simulink model "RateGyroUsingQuaternions"  (R2020b)
settings: Solver=VariableStepAuto  StartTime=0.0  StopTime=50  RelTol=1e-3
libraries: simulink_extras x1
settings Model: Creator=dariusmensah  LastModifiedBy=dariusmensah

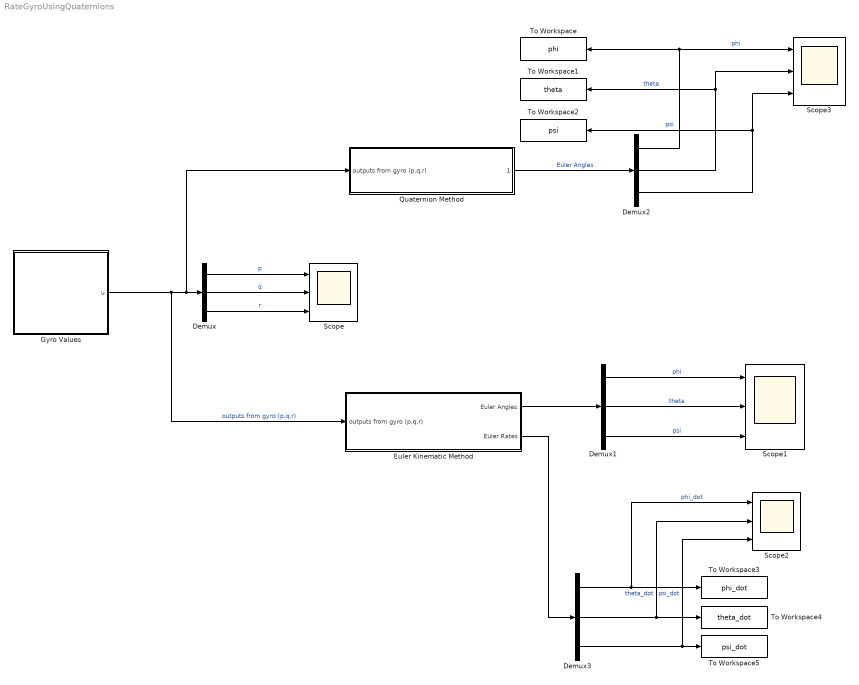
== system RateGyroUsingQuaternions ==
  Demux{,1..3} (4 alike) : Demux  Outputs=3
  Euler Kinematic Method : Subsystem
  Gyro Values : Subsystem
  Quaternion Method : Subsystem
  Scope{,1..3} (4 alike) : Scope  NumInputPorts=3
  To Workspace : ToWorkspace  VariableName=phi  SaveFormat=Structure With Time  SampleTime=-1
  To Workspace1 : ToWorkspace  VariableName=theta  SaveFormat=Structure With Time  SampleTime=-1
  To Workspace2 : ToWorkspace  VariableName=psi  SaveFormat=Structure With Time  SampleTime=-1
  To Workspace3 : ToWorkspace  VariableName=phi_dot  SaveFormat=Structure With Time  SampleTime=-1
  To Workspace4 : ToWorkspace  VariableName=theta_dot  SaveFormat=Structure With Time  SampleTime=-1
  To Workspace5 : ToWorkspace  VariableName=psi_dot  SaveFormat=Structure With Time  SampleTime=-1
  wires:
  Demux1/3 -> Scope1/3  "psi"
  Demux3/3 -> Scope2/3, To Workspace5/1  "psi_dot"
  Demux/3 -> Scope/3  "r"
  Gyro Values/1(u) -> Euler Kinematic Method/1(outputs from gyro (p,q,r)), Quaternion Method/1(outputs from gyro (p,q,r)), Demux/1  "outputs from gyro (p,q,r)"
  Demux/2 -> Scope/2  "q"
  Demux3/1 -> To Workspace3/1, Scope2/1  "phi_dot"
  Demux3/2 -> To Workspace4/1, Scope2/2  "theta_dot"
  Demux/1 -> Scope/1  "p"
  Demux1/1 -> Scope1/1  "phi"
  Demux1/2 -> Scope1/2  "theta"
  Quaternion Method/1(" ") -> Demux2/1  "Euler Angles"
  Demux2/1 -> To Workspace/1, Scope3/1  "phi"
  Demux2/2 -> Scope3/2, To Workspace1/1  "theta"
  Demux2/3 -> Scope3/3, To Workspace2/1  "psi"
  Euler Kinematic Method/1(Euler Angles) -> Demux1/1
  Euler Kinematic Method/2(Euler Rates) -> Demux3/1

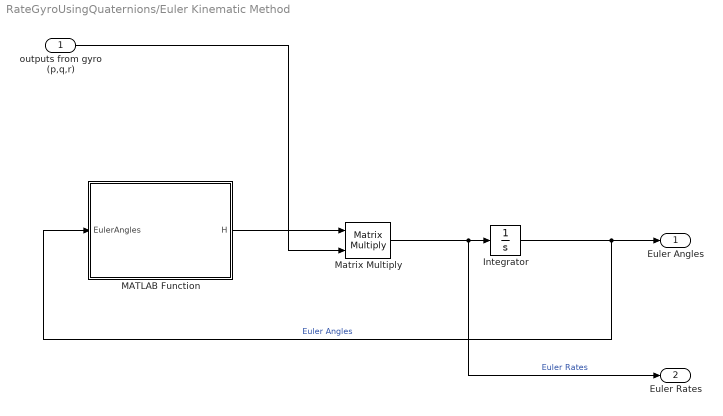
== system RateGyroUsingQuaternions/Euler Kinematic Method ==
  outputs from gyro (p,q,r) : Inport
  Integrator : Integrator  InitialCondition=[0;0;0]
  MATLAB Function : MATLAB Function  TreatAsAtomicUnit=on
  Matrix Multiply : Product  Multiplication=Matrix(*)
  Euler Angles : Outport
  Euler Rates : Outport  Port=2
  wires:
  outputs from gyro (p,q,r)/1 -> Matrix Multiply/2
  Integrator/1 -> Euler Angles/1, MATLAB Function/1(EulerAngles)  "Euler Angles"
  Matrix Multiply/1 -> Euler Rates/1, Integrator/1  "Euler Rates"
  MATLAB Function/1(H) -> Matrix Multiply/1

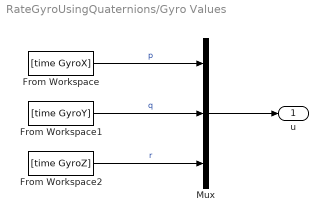
== system RateGyroUsingQuaternions/Gyro Values ==
  From Workspace : FromWorkspace  VariableName=[time GyroX]
  From Workspace1 : FromWorkspace  VariableName=[time GyroY]
  From Workspace2 : FromWorkspace  VariableName=[time GyroZ]
  Mux : Mux  Inputs=3
  u : Outport
  wires:
  From Workspace2/1 -> Mux/3  "r"
  From Workspace/1 -> Mux/1  "p"
  From Workspace1/1 -> Mux/2  "q"
  Mux/1 -> u/1

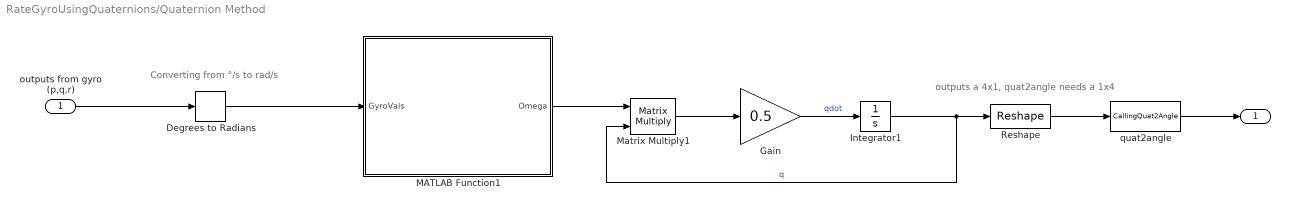
== system RateGyroUsingQuaternions/Quaternion Method ==
  note: outputs a 4x1, quat2angle needs a 1x4
  note: Converting from °/s to rad/s
  outputs from gyro (p,q,r) : Inport
  " quat2angle" : MATLABFcn  MATLABFcn=CallingQuat2Angle
  Degrees to Radians : simulink_extras/Transformations/Degrees to Radians
  Gain : Gain  Gain=0.5
  Integrator1 : Integrator  InitialCondition=[1;0;0;0]
  MATLAB Function1 : MATLAB Function  TreatAsAtomicUnit=on
  Matrix Multiply1 : Product  Multiplication=Matrix(*)
  Reshape : Reshape  OutputDimensionality=Customize  OutputDimensions=[1,4]
  " " : Outport
  wires:
  " quat2angle"/1 -> " "/1
  outputs from gyro (p,q,r)/1 -> Degrees to Radians/1
  Gain/1 -> Integrator1/1  "qdot"
  Degrees to Radians/1 -> MATLAB Function1/1(GyroVals)
  Matrix Multiply1/1 -> Gain/1
  Integrator1/1 -> Reshape/1, Matrix Multiply1/2  "q"
  Reshape/1 -> " quat2angle"/1
  MATLAB Function1/1(Omega) -> Matrix Multiply1/1

== matlab function RateGyroUsingQuaternions/Euler Kinematic Method/MATLAB Function ==
  data: EulerAngles input; H output
function H = EulerKinematicEq (EulerAngles)

phi = EulerAngles(1);
theta = EulerAngles(2);


H = [1 sind(phi)*tand(theta) -cosd(phi)*tand(theta); 
       0 cosd(phi) sind(phi);
       0 -sind(phi)*secd(theta) cosd(phi)*secd(theta)];
end

== matlab function RateGyroUsingQuaternions/Quaternion Method/MATLAB Function1 ==
  data: GyroVals input; Omega output
function Omega = QuaternionDerivative(GyroVals)

gyroX = GyroVals(1);
gyroY = GyroVals(2);
gyroZ = GyroVals(3);

Omega = [0 -gyroX -gyroY -gyroZ;
        gyroX 0 gyroZ -gyroY;
        gyroY -gyroZ 0 gyroX;
        gyroZ gyroY -gyroX 0];
end
